simulink model "modele_V6"  (R2025b)
settings: Solver=FixedStepDiscrete  StartTime=0.0  StopTime=10  FixedStep=0.005  RelTol=1e-3
values from neighbouring files (symbols this model uses):
  kalman_data = design_Kalman(p)    [checker.m]    (also in export_gains_to_c.m; main_simu.m)
  lqi_data = design_LQI(p)    [checker.m]    (also in export_gains_to_c.m)
  mpc_data = rmfield(mpc_data, {'P_osqp', 'A_osqp'})    [build_osqp_solver.m]    (also in checker.m; export_gains_to_c.m = design_MPC(p); main_simu.m)
  p = load_parameters()    [build_osqp_solver.m]    (also in checker.m; export_gains_to_c.m)
undefined symbols (not defined in the file or in its folder): DiscIntNeverNeededParam, dspblkCoreblockFVToolHelper, gcbh
libraries: simulink x5
settings Model: Creator=THOMAS  LastModifiedBy=THOMAS
settings SFSimCC: SimUserSources=MahonyAHRS\MahonyAHRS.c  SimUserIncludeDirs=C:\Users\thoma\Desktop\ONERA\V4\MahonyAHRS  CustomCodeUndefinedFunction=DoNotDetect
settings SFSimCC: SimCustomHeaderCode=|
  | #include "MahonyAHRS.h"
  | extern volatile float q0, q1, q2, q3;
  | extern volatile float integralFBx, integralFBy, integralFBz;
settings RTWCC: RTWUseSimCustomCode=on  CustomInclude=C:\Users\thoma\Desktop\ONERA\V4\MahonyAHRS  CustomSource=MahonyAHRS\MahonyAHRS.c  Toolchain=MinGW64 | CMake/gmake (64-bit Windows)  BuildConfiguration=Release
settings RTWCC: CustomHeaderCode=|
  | #include "MahonyAHRS.h"
  | extern volatile float q0, q1, q2, q3;
  | extern volatile float integralFBx, integralFBy, integralFBz;

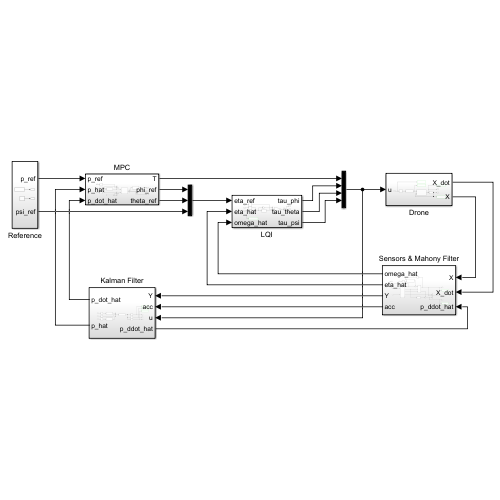
[thumbnail: Simulink's stored preview of the top-level diagram]
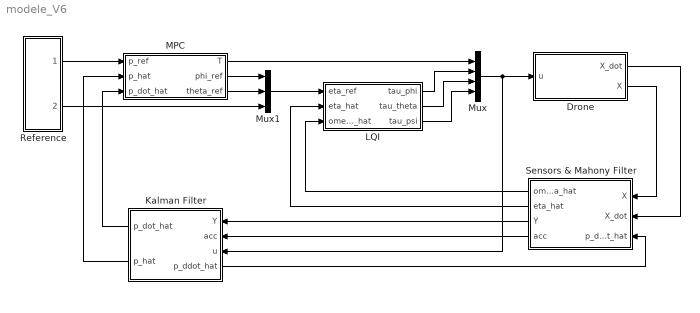
== system modele_V6 ==
  Drone : Subsystem
  Kalman Filter : Subsystem
      settings: PortSchema="{\"entries\":[{\"content\":{\"sides\":[{\"content\":{\"connectorIds\":[\"In1\",\"In2\",\"In3\",\"Out3\"]},\"type\":\"ConnectorPlacement.EquallySpacedRectSide\",\"uuid\":\"d1b80e43-277a-425d-bfea-a46540c59ade\"},{\"content\":{\"connectorIds\":[\"Out1\",\"Out2\"],\"side\":\"RIGHT\"},\"type\":\"ConnectorPlacement.EquallySpacedRectSide\",\"uuid\":\"e2b5c73d-e18d-4d88-8a3a-b4b6637fab46\"},{\"content\":{\"side\":\"TOP\"},\"type\":\"ConnectorPlacement.EquallySpacedRectSide\",\"uuid\":\"def8a2c3-4beb-4693-b110-6586be4b0baf\"}]},\"type\":\"ConnectorPlacement.EquallySpacedConnector\",\"uuid\":\"a4526f81-9c75-4300-957b-6f8428e841a4\"}],\"packageUris\":[\"http://schema.mathworks.com/mf0/Connector/R2020b\"],\"version\":\"1.0\"}"
  LQI : Subsystem
  MPC : Subsystem
  Mux : Mux
  Mux1 : Mux  Inputs=3
  Reference : Subsystem
  Sensors & Mahony Filter : Subsystem
  wires:
  Mux/1 -> Drone/1(u), Kalman Filter/3(u)
  LQI/1(tau_phi) -> Mux/2
  LQI/2(tau_theta) -> Mux/3
  LQI/3(tau_psi) -> Mux/4
  Reference/1(p_ref) -> MPC/1(p_ref)
  Mux1/1 -> LQI/1(eta_ref)
  Reference/2(psi_ref) -> Mux1/3
  Kalman Filter/2(p_hat) -> MPC/2(p_hat)
  Drone/2(X) -> Sensors & Mahony Filter/1(X)
  Kalman Filter/1(p_dot_hat) -> MPC/3(p_dot_hat)
  Sensors & Mahony Filter/3(Y) -> Kalman Filter/1(Y)
  Drone/1(X_dot) -> Sensors & Mahony Filter/2(X_dot)
  Sensors & Mahony Filter/2(eta_hat) -> LQI/2(eta_hat)
  Sensors & Mahony Filter/1(omega_hat) -> LQI/3(omega_hat)
  MPC/3(theta_ref) -> Mux1/2
  MPC/2(phi_ref) -> Mux1/1
  Sensors & Mahony Filter/4(acc) -> Kalman Filter/2(acc)
  Kalman Filter/3(p_ddot_hat) -> Sensors & Mahony Filter/3(p_ddot_hat)
  MPC/1(T) -> Mux/1

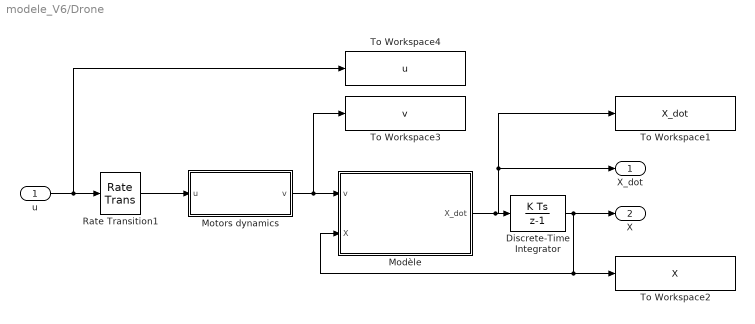
== system modele_V6/Drone ==
  u : Inport
  Discrete-Time Integrator : DiscreteIntegrator  SampleTime=1/p.f_plant  ICPrevOutput=DiscIntNeverNeededParam  ICPrevScaledInput=DiscIntNeverNeededParam
  Modèle : MATLAB Function  TreatAsAtomicUnit=on
  Motors dynamics : Subsystem
  Rate Transition1 : RateTransition  InitialCondition=[p.M*p.g; 0; 0; 0]  OutPortSampleTime=1/p.f_plant
  To Workspace1 : ToWorkspace  VariableName=X_dot  SaveFormat=Timeseries  SampleTime=-1
  To Workspace2 : ToWorkspace  VariableName=X  SaveFormat=Timeseries  SampleTime=-1
  To Workspace3 : ToWorkspace  VariableName=v  SaveFormat=Timeseries  SampleTime=-1
  To Workspace4 : ToWorkspace  VariableName=u  SaveFormat=Timeseries  SampleTime=-1
  X_dot : Outport
  X : Outport  Port=2
  wires:
  Modèle/1(X_dot) -> X_dot/1, To Workspace1/1, Discrete-Time Integrator/1
  Discrete-Time Integrator/1 -> X/1, Modèle/2(X), To Workspace2/1
  u/1 -> To Workspace4/1, Rate Transition1/1
  Motors dynamics/1(v) -> To Workspace3/1, Modèle/1(v)
  Rate Transition1/1 -> Motors dynamics/1(u)

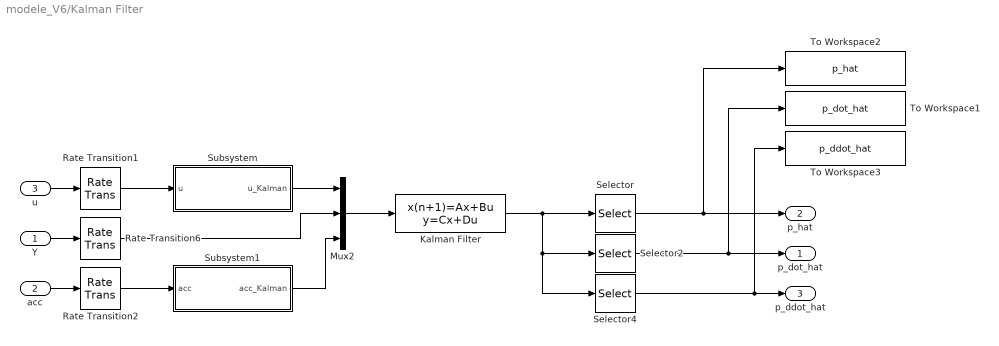
== system modele_V6/Kalman Filter ==
  Y : Inport
  acc : Inport  Port=2
  u : Inport  Port=3
  Kalman Filter : DiscreteStateSpace  A=kalman_data.sys_d.a - kalman_data.K*kalman_data.sys_d.c  B=[kalman_data.sys_d.b kalman_data.K]  C=eye(15)  D=zeros(15, 16)  SampleTime=1/p.f_kalman
  Mux2 : Mux  Inputs=3
  Rate Transition1 : RateTransition  OutPortSampleTime=1/p.f_kalman
  Rate Transition2 : RateTransition  OutPortSampleTime=1/p.f_kalman
  Rate Transition6 : RateTransition  OutPortSampleTime=1/p.f_kalman
  Selector : Selector  InputPortWidth=15  IndexOptions=Index vector (dialog)  Indices=[1:3]  OutputSizes=1
  Selector2 : Selector  InputPortWidth=15  IndexOptions=Index vector (dialog)  Indices=[7:9]  OutputSizes=1
  Selector4 : Selector  InputPortWidth=15  IndexOptions=Index vector (dialog)  Indices=[13:15]  OutputSizes=1
  Subsystem : Subsystem
  Subsystem1 : Subsystem
  To Workspace1 : ToWorkspace  VariableName=p_dot_hat  SaveFormat=Timeseries  SampleTime=-1
  To Workspace2 : ToWorkspace  VariableName=p_hat  SaveFormat=Timeseries  SampleTime=-1
  To Workspace3 : ToWorkspace  VariableName=p_ddot_hat  SaveFormat=Timeseries  SampleTime=-1
  p_dot_hat : Outport
  p_hat : Outport  Port=2
  p_ddot_hat : Outport  Port=3
  wires:
  Mux2/1 -> Kalman Filter/1
  Subsystem/1(u_Kalman) -> Mux2/1
  u/1 -> Rate Transition1/1
  Selector2/1 -> To Workspace1/1, p_dot_hat/1
  Kalman Filter/1 -> Selector4/1, Selector2/1, Selector/1
  Selector/1 -> p_hat/1, To Workspace2/1
  Y/1 -> Rate Transition6/1
  Rate Transition6/1 -> Mux2/2
  Rate Transition1/1 -> Subsystem/1(u)
  acc/1 -> Rate Transition2/1
  Rate Transition2/1 -> Subsystem1/1(acc)
  Selector4/1 -> To Workspace3/1, p_ddot_hat/1
  Subsystem1/1(acc_Kalman) -> Mux2/3

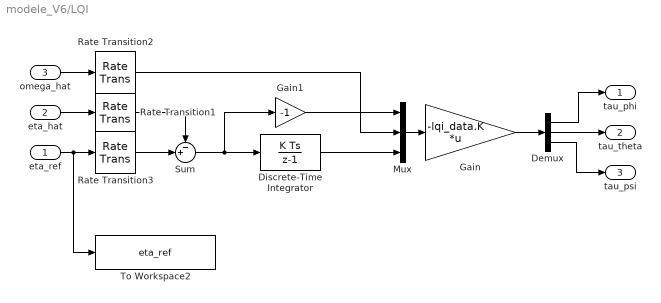
== system modele_V6/LQI ==
  eta_ref : Inport
  eta_hat : Inport  Port=2
  omega_hat : Inport  Port=3
  Demux : Demux  Outputs=3
  Discrete-Time Integrator : DiscreteIntegrator  SampleTime=1/p.f_lqi  ICPrevOutput=DiscIntNeverNeededParam  ICPrevScaledInput=DiscIntNeverNeededParam
  Gain : Gain  Gain=-lqi_data.K  Multiplication=Matrix(K*u)
  Gain1 : Gain  Gain=-1
  Mux : Mux  Inputs=3
  Rate Transition1 : RateTransition  OutPortSampleTime=1/p.f_lqi
  Rate Transition2 : RateTransition  OutPortSampleTime=1/p.f_lqi
  Rate Transition3 : RateTransition  OutPortSampleTime=1/p.f_lqi
  Sum : Sum  Inputs=-+|
  To Workspace2 : ToWorkspace  VariableName=eta_ref  SaveFormat=Timeseries  SampleTime=-1
  tau_phi : Outport
  tau_theta : Outport  Port=2
  tau_psi : Outport  Port=3
  wires:
  Gain/1 -> Demux/1
  Mux/1 -> Gain/1
  Discrete-Time Integrator/1 -> Mux/3
  omega_hat/1 -> Rate Transition2/1
  eta_hat/1 -> Rate Transition1/1
  eta_ref/1 -> To Workspace2/1, Rate Transition3/1
  Sum/1 -> Gain1/1, Discrete-Time Integrator/1
  Demux/1 -> tau_phi/1
  Demux/2 -> tau_theta/1
  Demux/3 -> tau_psi/1
  Rate Transition3/1 -> Sum/2
  Rate Transition2/1 -> Mux/2
  Rate Transition1/1 -> Sum/1
  Gain1/1 -> Mux/1

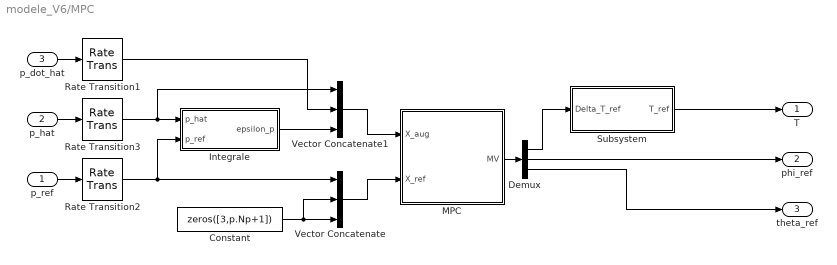
== system modele_V6/MPC ==
  p_ref : Inport
  p_hat : Inport  Port=2
  p_dot_hat : Inport  Port=3
  Constant : Constant  Value=zeros([3,p.Np+1])
  Demux : Demux  Outputs=3
  Integrale : Subsystem
  MPC : Subsystem
  Rate Transition1 : RateTransition  OutPortSampleTime=1/p.f_mpc
  Rate Transition2 : RateTransition  OutPortSampleTime=1/p.f_mpc
  Rate Transition3 : RateTransition  OutPortSampleTime=1/p.f_mpc
  Subsystem : Subsystem
  Vector Concatenate : Concatenate  NumInputs=3  Mode=Multidimensional array
  Vector Concatenate1 : Concatenate  NumInputs=3  Mode=Multidimensional array
  T : Outport
  phi_ref : Outport  Port=2
  theta_ref : Outport  Port=3
  wires:
  Vector Concatenate1/1 -> MPC/1(X_aug)
  MPC/1(MV) -> Demux/1
  Demux/1 -> Subsystem/1(Delta_T_ref)
  Integrale/1(epsilon_p) -> Vector Concatenate1/3
  Vector Concatenate/1 -> MPC/2(X_ref)
  Constant/1 -> Vector Concatenate/2, Vector Concatenate/3
  p_hat/1 -> Rate Transition3/1
  p_dot_hat/1 -> Rate Transition1/1
  Rate Transition3/1 -> Vector Concatenate1/1, Integrale/1(p_hat)
  p_ref/1 -> Rate Transition2/1
  Rate Transition1/1 -> Vector Concatenate1/2
  Demux/2 -> phi_ref/1
  Demux/3 -> theta_ref/1
  Rate Transition2/1 -> Vector Concatenate/1, Integrale/2(p_ref)
  Subsystem/1(T_ref) -> T/1

== system modele_V6/Reference ==
  Constant : Constant  Value=0
  From Workspace : FromWorkspace  VariableName=ref
  p_ref : Outport
  psi_ref : Outport  Port=2
  wires:
  Constant/1 -> psi_ref/1
  From Workspace/1 -> p_ref/1

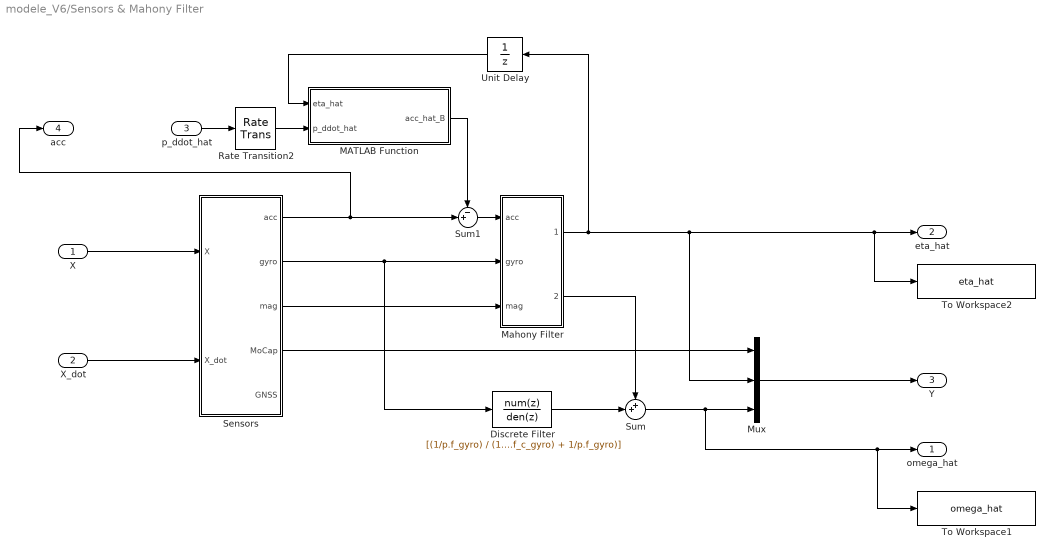
== system modele_V6/Sensors & Mahony Filter ==
  X : Inport
  X_dot : Inport  Port=2
  p_ddot_hat : Inport  Port=3
  Discrete Filter : DiscreteFilter  LoadFcn=dspblkCoreblockFVToolHelper(gcbh,'load');  Numerator=[(1/p.f_gyro) / (1/(2*pi*p.f_c_gyro) + 1/p.f_gyro)]  Denominator=[1, -1/(2*pi*p.f_c_gyro) / (1/(2*pi*p.f_c_gyro) + 1/p.f_gyro)]
      settings: CopyFcn=dspblkCoreblockFVToolHelper(gcbh,'copy');  DeleteFcn=dspblkCoreblockFVToolHelper(gcbh,'close');  ModelCloseFcn=dspblkCoreblockFVToolHelper(gcbh,'close');  PreSaveFcn=dspblkCoreblockFVToolHelper(gcbh,'presave');  PostSaveFcn=dspblkCoreblockFVToolHelper(gcbh,'postsave');  CloseFcn=dspblkCoreblockFVToolHelper(gcbh,'close');
  MATLAB Function : MATLAB Function  TreatAsAtomicUnit=on
  Mahony Filter : Subsystem
  Mux : Mux  Inputs=3
  Rate Transition2 : RateTransition  OutPortSampleTime=1/p.f_mahony
  Sensors : Subsystem
  Sum : Sum  Inputs=++|
  Sum1 : Sum  Inputs=-+|
  To Workspace1 : ToWorkspace  VariableName=omega_hat  SaveFormat=Timeseries  SampleTime=-1
  To Workspace2 : ToWorkspace  VariableName=eta_hat  SaveFormat=Timeseries  SampleTime=-1
  Unit Delay : UnitDelay  SampleTime=1/p.f_mahony  HasFrameUpgradeWarning=on
  omega_hat : Outport
  eta_hat : Outport  Port=2
  Y : Outport  Port=3
  acc : Outport  Port=4
  wires:
  X/1 -> Sensors/1(X)
  X_dot/1 -> Sensors/2(X_dot)
  Sensors/2(gyro) -> Discrete Filter/1, Mahony Filter/2(gyro)
  Mahony Filter/1(eta_hat) -> Mux/2, To Workspace2/1, eta_hat/1, Unit Delay/1
  Mux/1 -> Y/1
  Sensors/3(mag) -> Mahony Filter/3(mag)
  Sum/1 -> To Workspace1/1, omega_hat/1, Mux/3
  Mahony Filter/2(bias_hat) -> Sum/1
  Discrete Filter/1 -> Sum/2
  Sensors/4(MoCap) -> Mux/1
  Sum1/1 -> Mahony Filter/1(acc)
  Rate Transition2/1 -> MATLAB Function/2(p_ddot_hat)
  MATLAB Function/1(acc_hat_B) -> Sum1/1
  p_ddot_hat/1 -> Rate Transition2/1
  Unit Delay/1 -> MATLAB Function/1(eta_hat)
  Sensors/1(acc) -> Sum1/2, acc/1

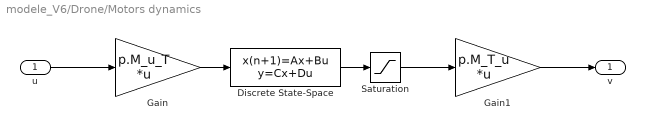
== system modele_V6/Drone/Motors dynamics ==
  u : Inport
  Discrete State-Space : DiscreteStateSpace  A=exp(-1/p.f_plant/p.tau_m) * eye(4)  B=(1 - exp(-1/p.f_plant/p.tau_m)) * eye(4)  C=eye(4)  D=zeros(4)  InitialCondition=ones(4,1)*p.M*p.g/4  SampleTime=1/p.f_plant
  Gain : Gain  Gain=p.M_u_T  Multiplication=Matrix(K*u)
  Gain1 : Gain  Gain=p.M_T_u  Multiplication=Matrix(K*u)
  Saturation : Saturate  UpperLimit=ones(4,1)*p.Ti_max  LowerLimit=ones(4,1)*p.Ti_min
  v : Outport
  wires:
  u/1 -> Gain/1
  Gain1/1 -> v/1
  Saturation/1 -> Gain1/1
  Discrete State-Space/1 -> Saturation/1
  Gain/1 -> Discrete State-Space/1

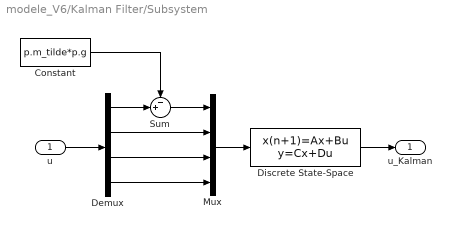
== system modele_V6/Kalman Filter/Subsystem ==
  u : Inport
  Constant : Constant  Value=p.m_tilde*p.g
  Demux : Demux
  Discrete State-Space : DiscreteStateSpace  A=exp(-1/p.f_kalman/p.tau_m) * eye(4)  B=(1 - exp(-1/p.f_kalman/p.tau_m)) * eye(4)  C=eye(4)  D=zeros(4)  SampleTime=1/p.f_kalman
  Mux : Mux
  Sum : Sum  Inputs=-+|
  u_Kalman : Outport
  wires:
  Constant/1 -> Sum/1
  Demux/1 -> Sum/2
  u/1 -> Demux/1
  Sum/1 -> Mux/1
  Demux/2 -> Mux/2
  Demux/3 -> Mux/3
  Demux/4 -> Mux/4
  Mux/1 -> Discrete State-Space/1
  Discrete State-Space/1 -> u_Kalman/1

== system modele_V6/Kalman Filter/Subsystem1 ==
  acc : Inport
  Bias : Bias  Bias=-p.g  SaturateOnIntegerOverflow=off
  Demux : Demux  Outputs=3
  Mux : Mux  Inputs=3
  acc_Kalman : Outport
  wires:
  Mux/1 -> acc_Kalman/1
  acc/1 -> Demux/1
  Demux/1 -> Mux/1
  Demux/2 -> Mux/2
  Demux/3 -> Bias/1
  Bias/1 -> Mux/3

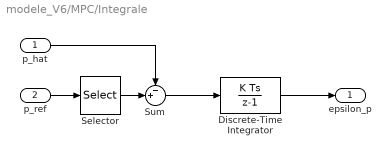
== system modele_V6/MPC/Integrale ==
  p_hat : Inport
  p_ref : Inport  Port=2
  Discrete-Time Integrator : DiscreteIntegrator  SampleTime=1/p.f_mpc  ICPrevOutput=DiscIntNeverNeededParam  ICPrevScaledInput=DiscIntNeverNeededParam
  Selector : Selector  NumberOfDimensions=2  InputPortWidth=16  IndexOptions=Index vector (dialog),Index vector (dialog)  Indices=[1:3],1  OutputSizes=1,1
  Sum : Sum  Inputs=-+|
  epsilon_p : Outport
  wires:
  p_ref/1 -> Selector/1
  p_hat/1 -> Sum/1
  Discrete-Time Integrator/1 -> epsilon_p/1
  Selector/1 -> Sum/2
  Sum/1 -> Discrete-Time Integrator/1

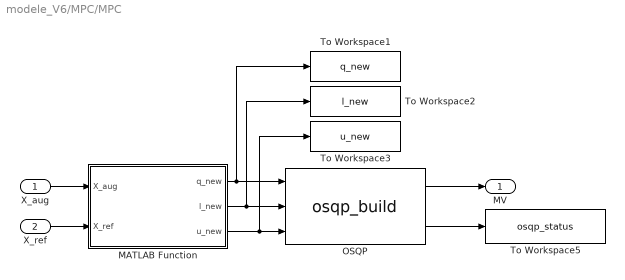
== system modele_V6/MPC/MPC ==
  X_aug : Inport
  X_ref : Inport  Port=2
  MATLAB Function : MATLAB Function  TreatAsAtomicUnit=on
  OSQP : S-Function  FunctionName=osqp_build  SFunctionDeploymentMode=off  EnableBusSupport=off
  To Workspace1 : ToWorkspace  VariableName=q_new  SaveFormat=Timeseries  SampleTime=-1
  To Workspace2 : ToWorkspace  VariableName=l_new  SaveFormat=Timeseries  SampleTime=-1
  To Workspace3 : ToWorkspace  VariableName=u_new  SaveFormat=Timeseries  SampleTime=-1
  To Workspace5 : ToWorkspace  VariableName=osqp_status  SaveFormat=Timeseries  SampleTime=-1
  MV : Outport
  wires:
  MATLAB Function/3(u_new) -> OSQP/3, To Workspace3/1
  MATLAB Function/2(l_new) -> OSQP/2, To Workspace2/1
  MATLAB Function/1(q_new) -> OSQP/1, To Workspace1/1
  OSQP/1 -> MV/1
  OSQP/2 -> To Workspace5/1
  X_aug/1 -> MATLAB Function/1(X_aug)
  X_ref/1 -> MATLAB Function/2(X_ref)

== system modele_V6/MPC/Subsystem ==
  Delta_T_ref : Inport
  Constant : Constant  Value=p.m_tilde*p.g
  Sum : Sum  Inputs=++|
  T_ref : Outport
  wires:
  Sum/1 -> T_ref/1
  Delta_T_ref/1 -> Sum/2
  Constant/1 -> Sum/1

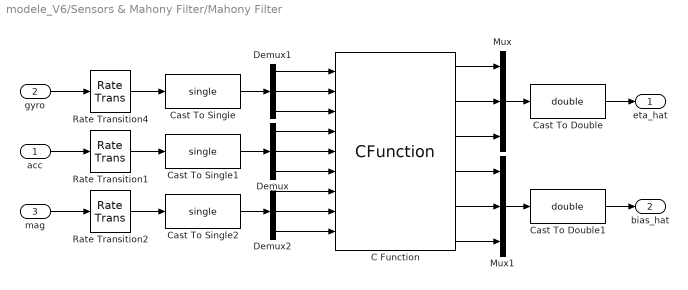
== system modele_V6/Sensors & Mahony Filter/Mahony Filter ==
  acc : Inport
  gyro : Inport  Port=2
  mag : Inport  Port=3
  C Function : CFunction  OutputCode=|  InitializeConditionsCode=|  CodegenOutputCode=|  CodegenInitializeConditionsCode=|  SampleTime=1/p.f_mahony  CustomCodeSettingLocation=ModelConfigurationParameters
      OutputCode=|
      | MahonyAHRSupdate(gx, gy, gz, ax, ay, az, mx, my, mz);
      | getEulerAngles(&roll, &pitch, &yaw);
      | MahonyAHRSgetBias(&bx, &by, &bz);
      InitializeConditionsCode=|
      | q0 = 1.0f;
      | q1 = 0.0f;
      | q2 = 0.0f;
      | q3 = 0.0f;
      | 
      | integralFBx = 0.0f;
      | integralFBy = 0.0f;
      | integralFBz = 0.0f;
      CodegenOutputCode=|
      | MahonyAHRSupdate(gx, gy, gz, ax, ay, az, mx, my, mz);
      | getEulerAngles(&roll, &pitch, &yaw);
      | MahonyAHRSgetBias(&bx, &by, &bz);
      CodegenInitializeConditionsCode=|
      | q0 = 1.0f;
      | q1 = 0.0f;
      | q2 = 0.0f;
      | q3 = 0.0f;
      | 
      | integralFBx = 0.0f;
      | integralFBy = 0.0f;
      | integralFBz = 0.0f;
  Cast To Double : DataTypeConversion  OutDataTypeStr=double  SaturateOnIntegerOverflow=off  RndMeth=Floor
  Cast To Double1 : DataTypeConversion  OutDataTypeStr=double  SaturateOnIntegerOverflow=off  RndMeth=Floor
  Cast To Single : DataTypeConversion  OutDataTypeStr=single  SaturateOnIntegerOverflow=off  RndMeth=Floor
  Cast To Single1 : DataTypeConversion  OutDataTypeStr=single  SaturateOnIntegerOverflow=off  RndMeth=Floor
  Cast To Single2 : DataTypeConversion  OutDataTypeStr=single  SaturateOnIntegerOverflow=off  RndMeth=Floor
  Demux : Demux  Outputs=3
  Demux1 : Demux  Outputs=3
  Demux2 : Demux  Outputs=3
  Mux : Mux  Inputs=3
  Mux1 : Mux  Inputs=3
  Rate Transition1 : RateTransition  OutPortSampleTime=1/p.f_mahony
  Rate Transition2 : RateTransition  OutPortSampleTime=1/p.f_mahony
  Rate Transition4 : RateTransition  OutPortSampleTime=1/p.f_mahony
  eta_hat : Outport
  bias_hat : Outport  Port=2
  wires:
  Demux/3 -> C Function/6
  Demux/2 -> C Function/5
  Demux/1 -> C Function/4
  acc/1 -> Rate Transition1/1
  Demux1/3 -> C Function/3
  Demux1/1 -> C Function/1
  Demux1/2 -> C Function/2
  gyro/1 -> Rate Transition4/1
  C Function/3 -> Mux/3
  C Function/2 -> Mux/2
  C Function/1 -> Mux/1
  Mux/1 -> Cast To Double/1
  Cast To Single/1 -> Demux1/1
  Cast To Single1/1 -> Demux/1
  Cast To Double/1 -> eta_hat/1
  Cast To Single2/1 -> Demux2/1
  Demux2/3 -> C Function/9
  Demux2/2 -> C Function/8
  mag/1 -> Rate Transition2/1
  Demux2/1 -> C Function/7
  C Function/4 -> Mux1/1
  C Function/5 -> Mux1/2
  C Function/6 -> Mux1/3
  Mux1/1 -> Cast To Double1/1
  Cast To Double1/1 -> bias_hat/1
  Rate Transition4/1 -> Cast To Single/1
  Rate Transition1/1 -> Cast To Single1/1
  Rate Transition2/1 -> Cast To Single2/1

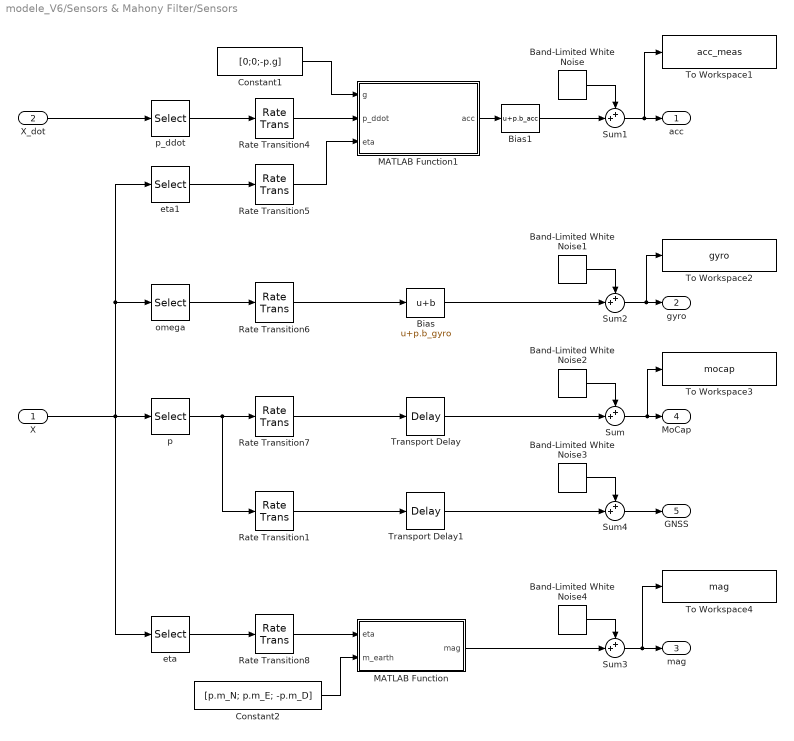
== system modele_V6/Sensors & Mahony Filter/Sensors ==
  X : Inport
  X_dot : Inport  Port=2
  Band-Limited White Noise : simulink/Sources/Band-Limited White Noise  Cov=p.sigma_acc^2/p.f_acc  Ts=1/p.f_acc  seed=[23341]
  Band-Limited White Noise1 : simulink/Sources/Band-Limited White Noise  Cov=p.sigma_omega^2/p.f_gyro  Ts=1/p.f_gyro  seed=[23341]
  Band-Limited White Noise2 : simulink/Sources/Band-Limited White Noise  Cov=p.sigma_p^2/p.f_MoCap  Ts=1/p.f_MoCap  seed=[23341]
  Band-Limited White Noise3 : simulink/Sources/Band-Limited White Noise  Cov=[p.sigma_p_xy^2/p.f_GNSS; p.sigma_p_xy^2/p.f_GNSS; p.sigma_p_z^2/p.f_GNSS]  Ts=1/p.f_GNSS  seed=[23341]
  Band-Limited White Noise4 : simulink/Sources/Band-Limited White Noise  Cov=p.sigma_mag^2/p.f_mag  Ts=1/p.f_mag  seed=[23341]
  Bias : Bias  Bias=p.b_gyro  SaturateOnIntegerOverflow=off
  Bias1 : Bias  Bias=p.b_acc  SaturateOnIntegerOverflow=off
  Constant1 : Constant  Value=[0;0;-p.g]
  Constant2 : Constant  Value=[p.m_N; p.m_E; -p.m_D]
  MATLAB Function : MATLAB Function  TreatAsAtomicUnit=on
  MATLAB Function1 : MATLAB Function  TreatAsAtomicUnit=on
  Rate Transition1 : RateTransition  OutPortSampleTime=1/p.f_GNSS
  Rate Transition4 : RateTransition  OutPortSampleTime=1/p.f_acc
  Rate Transition5 : RateTransition  OutPortSampleTime=1/p.f_acc
  Rate Transition6 : RateTransition  OutPortSampleTime=1/p.f_gyro
  Rate Transition7 : RateTransition  OutPortSampleTime=1/p.f_MoCap
  Rate Transition8 : RateTransition  OutPortSampleTime=1/p.f_mag
  Sum{,1..4} (5 alike) : Sum  Inputs=++|
  To Workspace1 : ToWorkspace  VariableName=acc_meas  SaveFormat=Timeseries  SampleTime=-1
  To Workspace2 : ToWorkspace  VariableName=gyro  SaveFormat=Timeseries  SampleTime=-1
  To Workspace3 : ToWorkspace  VariableName=mocap  SaveFormat=Timeseries  SampleTime=-1
  To Workspace4 : ToWorkspace  VariableName=mag  SaveFormat=Timeseries  SampleTime=-1
  Transport Delay : TransportDelay  DelayTime=p.latency_MoCap
  Transport Delay1 : TransportDelay  DelayTime=p.latency_GNSS
  eta : Selector  InputPortWidth=12  IndexOptions=Index vector (dialog)  Indices=[4:6]  OutputSizes=1
  eta1 : Selector  InputPortWidth=12  IndexOptions=Index vector (dialog)  Indices=[4:6]  OutputSizes=1
  omega : Selector  InputPortWidth=12  IndexOptions=Index vector (dialog)  Indices=[10:12]  OutputSizes=1
  p : Selector  InputPortWidth=12  IndexOptions=Index vector (dialog)  Indices=[1:3]  OutputSizes=1
  p_ddot : Selector  InputPortWidth=12  IndexOptions=Index vector (dialog)  Indices=[7:9]  OutputSizes=1
  acc : Outport
  gyro : Outport  Port=2
  mag : Outport  Port=3
  MoCap : Outport  Port=4
  GNSS : Outport  Port=5
  wires:
  X/1 -> eta/1, eta1/1, omega/1, p/1
  Sum1/1 -> To Workspace1/1, acc/1
  Sum2/1 -> To Workspace2/1, gyro/1
  Sum/1 -> To Workspace3/1, MoCap/1
  MATLAB Function/1(mag) -> Sum3/2
  Sum3/1 -> To Workspace4/1, mag/1
  MATLAB Function1/1(acc) -> Bias1/1
  Constant1/1 -> MATLAB Function1/1(g)
  Band-Limited White Noise/1 -> Sum1/1
  Band-Limited White Noise1/1 -> Sum2/1
  Band-Limited White Noise2/1 -> Sum/1
  Band-Limited White Noise4/1 -> Sum3/1
  Constant2/1 -> MATLAB Function/2(m_earth)
  Bias/1 -> Sum2/2
  Transport Delay/1 -> Sum/2
  Transport Delay1/1 -> Sum4/2
  Rate Transition1/1 -> Transport Delay1/1
  Sum4/1 -> GNSS/1
  Band-Limited White Noise3/1 -> Sum4/1
  Rate Transition7/1 -> Transport Delay/1
  p/1 -> Rate Transition1/1, Rate Transition7/1
  Rate Transition6/1 -> Bias/1
  omega/1 -> Rate Transition6/1
  eta1/1 -> Rate Transition5/1
  Rate Transition5/1 -> MATLAB Function1/3(eta)
  p_ddot/1 -> Rate Transition4/1
  X_dot/1 -> p_ddot/1
  Rate Transition4/1 -> MATLAB Function1/2(p_ddot)
  Rate Transition8/1 -> MATLAB Function/1(eta)
  eta/1 -> Rate Transition8/1
  Bias1/1 -> Sum1/2

== matlab function modele_V6/Sensors & Mahony Filter/Sensors/MATLAB Function ==
  data: eta input; mag output; m_earth input; p parameter
function mag = mag(eta, m_earth, p)

phi = eta(1);
theta = eta(2);
psi = eta(3);

R_B = [cos(theta)*cos(psi) sin(phi)*sin(theta)*cos(psi)-cos(phi)*sin(psi) cos(phi)*sin(theta)*cos(psi)+sin(phi)*sin(psi);
       cos(theta)*sin(psi) sin(phi)*sin(theta)*sin(psi)+cos(phi)*cos(psi) cos(phi)*sin(theta)*sin(psi)-sin(phi)*cos(psi);
       -sin(theta) sin(phi)*cos(theta) cos(phi)*cos(theta)];

mag = p.A_mag * (R_B' * m_earth) + p.B_mag;

== matlab function modele_V6/Drone/Modèle ==
  data: v input; X_dot output; X input; p parameter
function X_dot = Modele(v, X, p)

% X = [x y z phi theta psi x_dot y_dot z_dot p q r]
% v = [T tau_phi tau_theta tau_psi]

eta = X(4:6);
p_dot = X(7:9);
omega = X(10:12);

eta = eta(:); p_dot = p_dot(:); omega = omega(:);

% relation
phi = eta(1);
theta = eta(2);
psi = eta(3);

T_eta = [1 sin(phi)*tan(theta) cos(phi)*tan(theta);
         0 cos(phi) -sin(phi);
         0 sin(phi)*sec(theta) cos(phi)*sec(theta)];

eta_dot = T_eta * omega;

R_B = [cos(theta)*cos(psi) sin(phi)*sin(theta)*cos(psi)-cos(phi)*sin(psi) cos(phi)*sin(theta)*cos(psi)+sin(phi)*sin(psi);
       cos(theta)*sin(psi) sin(phi)*sin(theta)*sin(psi)+cos(phi)*cos(psi) cos(phi)*sin(theta)*sin(psi)-sin(phi)*cos(psi);
       -sin(theta) sin(phi)*cos(theta) cos(phi)*cos(theta)];

a3 = [0 0 1]';

A = [p_dot; eta_dot; -p.g*a3; (p.Iy-p.Iz)/p.Ix*omega(2)*omega(3); (p.Iz-p.Ix)/p.Iy*omega(1)*omega(3); (p.Ix-p.Iy)/p.Iz*omega(1)*omega(2)];
B = [zeros([6,1]) zeros([6,3]);
     1/p.M*R_B(:,3) zeros([3,3]);
     zeros([3,1]) inv(p.I)];

X_dot = A + B*v;

== matlab function modele_V6/MPC/MPC/MATLAB Function ==
  data: X_aug input; q_new output; l_new output; u_new output; X_ref input; p parameter; mpc_data parameter
function [q_new,l_new,u_new]= iterationData(X_aug, X_ref, p, mpc_data)

q_new = [reshape(-diag(p.Q_mpc) * X_ref(:, 1:p.Np), [], 1); -mpc_data.Q_T* p.Wterminale * X_ref(:, p.Np+1); zeros(mpc_data.m * p.Nc, 1)];
l_new = [X_aug(:); zeros(mpc_data.n*p.Np, 1); repmat(p.X_min(:), p.Np+1, 1); repmat(p.U_min(:), p.Nc, 1)];
u_new = [X_aug(:); zeros(mpc_data.n*p.Np, 1); repmat(p.X_max(:), p.Np+1, 1); repmat(p.U_max(:), p.Nc, 1)];

== matlab function modele_V6/Sensors & Mahony Filter/Sensors/MATLAB Function1 ==
  data: g input; acc output; p_ddot input; eta input
function acc = acc(g, p_ddot, eta)
phi = eta(1);
theta = eta(2);
psi = eta(3);

R_B = [cos(theta)*cos(psi) sin(phi)*sin(theta)*cos(psi)-cos(phi)*sin(psi) cos(phi)*sin(theta)*cos(psi)+sin(phi)*sin(psi);
       cos(theta)*sin(psi) sin(phi)*sin(theta)*sin(psi)+cos(phi)*cos(psi) cos(phi)*sin(theta)*sin(psi)-sin(phi)*cos(psi);
       -sin(theta) sin(phi)*cos(theta) cos(phi)*cos(theta)];

acc = R_B' * (p_ddot - g); % considere que l'acc est placé au CG sinon ( acc = R_B'*(p_ddot - g) + omega_dot * rp + omega^2 * rp

== matlab function modele_V6/Sensors & Mahony Filter/MATLAB Function ==
  data: eta_hat input; p_ddot_hat input; acc_hat_B output
function acc_hat_B = local(eta_hat, p_ddot_hat)

phi = eta_hat(1);
theta = eta_hat(2);
psi = eta_hat(3);

R_B = [cos(theta)*cos(psi) sin(phi)*sin(theta)*cos(psi)-cos(phi)*sin(psi) cos(phi)*sin(theta)*cos(psi)+sin(phi)*sin(psi);
       cos(theta)*sin(psi) sin(phi)*sin(theta)*sin(psi)+cos(phi)*cos(psi) cos(phi)*sin(theta)*sin(psi)-sin(phi)*cos(psi);
       -sin(theta) sin(phi)*cos(theta) cos(phi)*cos(theta)];

acc_hat_B = R_B' * p_ddot_hat;
